simulink model "STM_SIMULINK_BLDC"  (R2022a)
settings: Solver=FixedStepAuto  StartTime=0.0  StopTime=10.0  FixedStep=0.001  RelTol=1e-3  EnableMultiTasking=on
InitFcn:
  | dataType = 'single';
  | 
  | motor.polePairs = 6;
  | motor.base_speed = 4000;
  | motor.base_freq = 266.6667;
  | max_rpm = 1000;
  | Ts = 1e-3;
undefined symbols (not defined in the file or in its folder): DiscIntNeverNeededParam
libraries: mcbcontrolslib x2
settings Model: ExtModeTrigDuration=10  Creator=s269684  LastModifiedBy=s269684
settings OptimizationCC: EnhancedBackFolding=on  PassReuseOutputArgsAs=Individual arguments  ZeroExternalMemoryAtStartup=off  ZeroInternalMemoryAtStartup=off  MaxStackSize=64  OptimizeBlockOrder=speed  DifferentSizesBufferReuse=on  OptimizationCustomize=off  EfficientTunableParamExpr=on
settings DebuggingCC: ParameterTunabilityLossMsg=error
settings HardwareCC: ProdBitPerPointer=32  ProdBitPerSizeT=32  ProdBitPerPtrDiffT=32  ProdLargestAtomicInteger=Long  ProdLargestAtomicFloat=Double  ProdWordSize=32  ProdLongLongMode=on  ProdHWDeviceType=ARM Compatible->ARM Cortex
settings SFSimCC: MATLABDynamicMemAlloc=off
settings RTWCC: SystemTargetFile=ert.tlc  HardwareBoard=STM32 Nucleo F302R8  TemplateMakefile=ert_default_tmf  Toolchain=GNU Tools for ARM Embedded Processors
settings CodeAppCC: ForceParamTrailComments=on  IgnoreCustomStorageClasses=off  OperatorAnnotations=on  SimulinkDataObjDesc=on  SFDataObjDesc=on  InsertBlockDesc=on
settings ERTTargetCC: ExtModeTransport=3  ExtModeStaticAlloc=on  ExtModeStaticAllocSize=1000  ExtModeMexFile=ext_xcp  ExtModeIntrfLevel=Level2 - Open

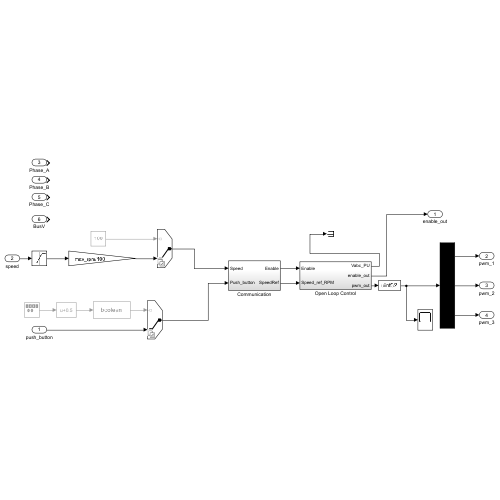
[thumbnail: Simulink's stored preview of the top-level diagram]
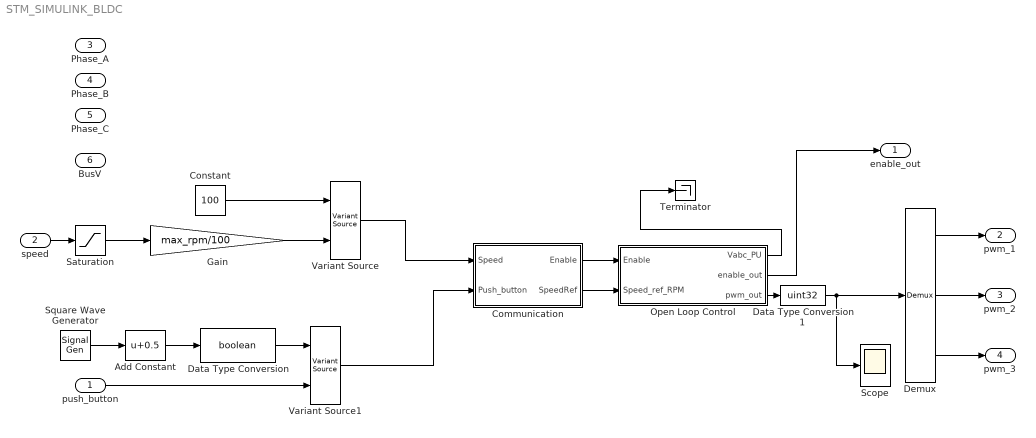
== system STM_SIMULINK_BLDC ==
  push_button : Inport  OutDataTypeStr=boolean
  speed : Inport  Port=2  OutDataTypeStr=uint16
  Phase_A : Inport  Port=3  OutDataTypeStr=uint16
  Phase_B : Inport  Port=4  OutDataTypeStr=uint16
  Phase_C : Inport  Port=5  OutDataTypeStr=uint16
  BusV : Inport  Port=6  OutDataTypeStr=uint16
  Add Constant : Bias  Bias=0.5  SaturateOnIntegerOverflow=off
  Communication : Subsystem
  Constant : Constant  Value=100  OutDataTypeStr=dataType
  Data Type Conversion : DataTypeConversion  OutDataTypeStr=boolean  SaturateOnIntegerOverflow=off  RndMeth=Floor
  Data Type Conversion1 : DataTypeConversion  OutDataTypeStr=uint32  SaturateOnIntegerOverflow=off  RndMeth=Floor
  Demux : Demux  Outputs=3
  Gain : Gain  Gain=max_rpm/100
  Open Loop Control : Subsystem
  Saturation : Saturate  UpperLimit=100  LowerLimit=0
  Scope : Scope
  Square Wave Generator : SignalGenerator  WaveForm=square  Amplitude=0.5  Frequency=0.5
  Terminator : Terminator
  Variant Source : VariantSource  VariantControlMode=sim codegen switching
  Variant Source1 : VariantSource  VariantControlMode=sim codegen switching
  enable_out : Outport
  pwm_1 : Outport  Port=2
  pwm_2 : Outport  Port=3
  pwm_3 : Outport  Port=4
  wires:
  Communication/2(SpeedRef) -> Open Loop Control/2(Speed_ref_RPM)
  Add Constant/1 -> Data Type Conversion/1
  Square Wave Generator/1 -> Add Constant/1
  Variant Source1/1 -> Communication/2(Push_button)
  Data Type Conversion/1 -> Variant Source1/1
  Saturation/1 -> Gain/1
  Open Loop Control/2(enable_out) -> enable_out/1
  speed/1 -> Saturation/1
  Demux/2 -> pwm_2/1
  Demux/1 -> pwm_1/1
  Open Loop Control/1(Vabc_PU) -> Terminator/1
  Communication/1(Enable) -> Open Loop Control/1(Enable)
  push_button/1 -> Variant Source1/2
  Variant Source/1 -> Communication/1(Speed)
  Data Type Conversion1/1 -> Scope/1, Demux/1
  Constant/1 -> Variant Source/1
  Open Loop Control/3(pwm_out) -> Data Type Conversion1/1
  Gain/1 -> Variant Source/2
  Demux/3 -> pwm_3/1

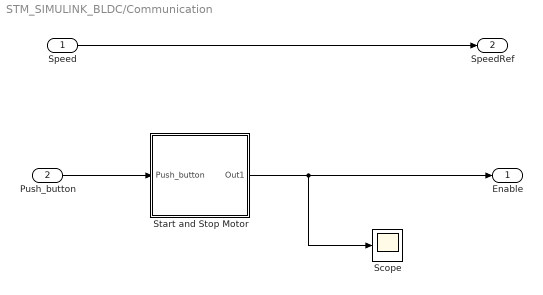
== system STM_SIMULINK_BLDC/Communication ==
  Speed : Inport
  Push_button : Inport  Port=2
  Scope : Scope
  Start and Stop Motor : Subsystem  TreatAsAtomicUnit=on  SystemSampleTime=1e-3
  Enable : Outport
  SpeedRef : Outport  Port=2  VectorParamsAs1DForOutWhenUnconnected=off
  wires:
  Speed/1 -> SpeedRef/1
  Start and Stop Motor/1(Out1) -> Scope/1, Enable/1
  Push_button/1 -> Start and Stop Motor/1(Push_button)

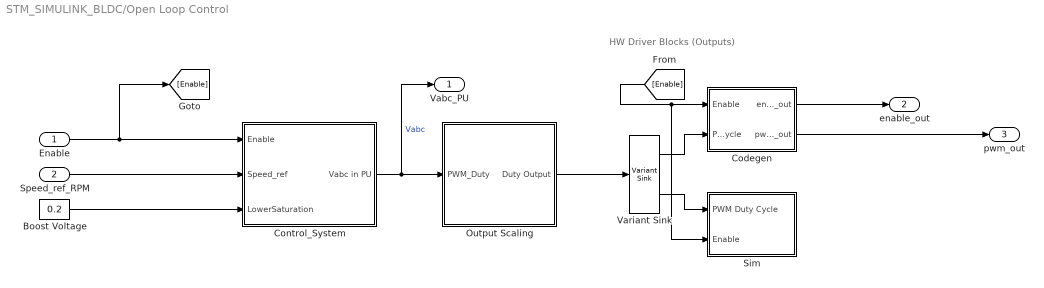
== system STM_SIMULINK_BLDC/Open Loop Control ==
  note: HW Driver Blocks (Outputs)
  Enable : Inport
  Speed_ref_RPM : Inport  Port=2
  Boost Voltage : Constant  Value=0.2  OutDataTypeStr=single
  Codegen : Subsystem
      settings: RTWSystemCode=Nonreusable function
  Control_System : Subsystem
      settings: RTWSystemCode=Nonreusable function
  Output Scaling : Subsystem
      settings: RTWSystemCode=Nonreusable function
  Sim : Subsystem
  Variant Sink : VariantSink  VariantControlMode=sim codegen switching
  Vabc_PU : Outport  VectorParamsAs1DForOutWhenUnconnected=off
  enable_out : Outport  Port=2
  pwm_out : Outport  Port=3
  wires:
  Control_System/1(Vabc in PU) -> Output Scaling/1(PWM_Duty), Vabc_PU/1  "Vabc"
  Boost Voltage/1 -> Control_System/3(LowerSaturation)
  Enable/1 -> [Enable], Control_System/1(Enable)
  Speed_ref_RPM/1 -> Control_System/2(Speed_ref)
  [Enable] -> Sim/2(Enable), Codegen/1(Enable)
  Variant Sink/1 -> Codegen/2(PWM Duty Cycle)
  Variant Sink/2 -> Sim/1(PWM Duty Cycle)
  Output Scaling/1(Duty Output) -> Variant Sink/1
  Codegen/1(enable_out) -> enable_out/1
  Codegen/2(pwm_out) -> pwm_out/1

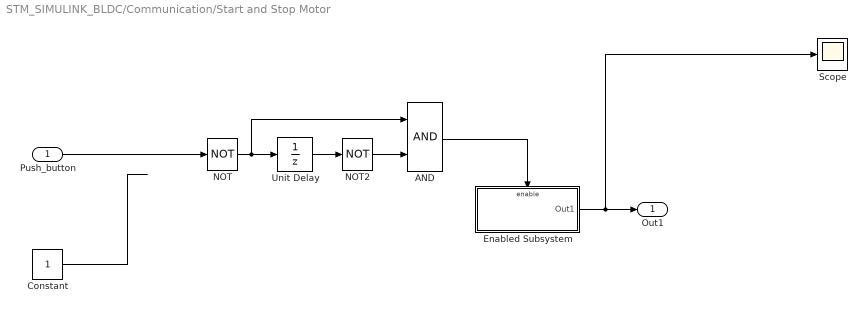
== system STM_SIMULINK_BLDC/Communication/Start and Stop Motor ==
  Push_button : Inport
  AND : Logic  AllPortsSameDT=off  OutDataTypeStr=boolean
  Constant : Constant  SampleTime=-1
  Enabled Subsystem : Subsystem  TreatAsAtomicUnit=on
  NOT : Logic  Operator=NOT  IconShape=distinctive  AllPortsSameDT=off  OutDataTypeStr=boolean
  NOT2 : Logic  Operator=NOT  IconShape=distinctive  AllPortsSameDT=off  OutDataTypeStr=boolean
  Scope : Scope
  Unit Delay : UnitDelay  InitialCondition=false  SampleTime=-1  HasFrameUpgradeWarning=on
  Out1 : Outport
  wires:
  Enabled Subsystem/1(Out1) -> Scope/1, Out1/1
  AND/1 -> Enabled Subsystem/Enable
  Push_button/1 -> NOT/1
  Unit Delay/1 -> NOT2/1
  NOT2/1 -> AND/2
  NOT/1 -> Unit Delay/1, AND/1
  Constant/1 -> ?

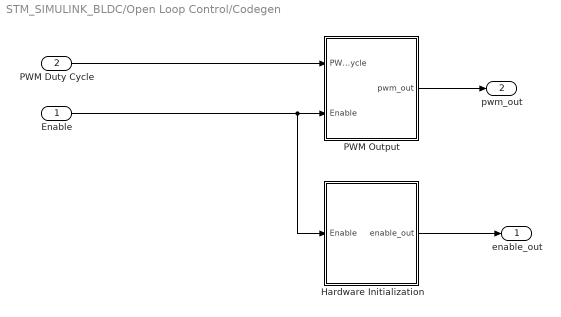
== system STM_SIMULINK_BLDC/Open Loop Control/Codegen ==
  Enable : Inport
  PWM Duty Cycle : Inport  Port=2
  Hardware Initialization : Subsystem
      settings: RTWSystemCode=Nonreusable function
  PWM Output : Subsystem
      settings: RTWSystemCode=Nonreusable function
  enable_out : Outport
  pwm_out : Outport  Port=2
  wires:
  PWM Duty Cycle/1 -> PWM Output/1(PWM Duty Cycle)
  Enable/1 -> Hardware Initialization/1(Enable), PWM Output/2(Enable)
  Hardware Initialization/1(enable_out) -> enable_out/1
  PWM Output/1(pwm_out) -> pwm_out/1

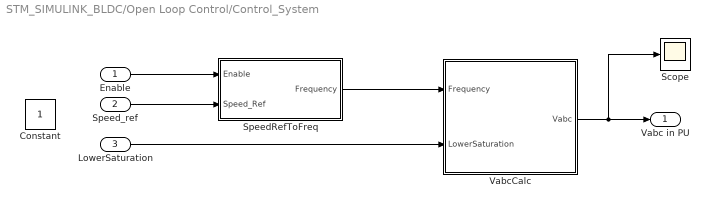
== system STM_SIMULINK_BLDC/Open Loop Control/Control_System ==
  Enable : Inport
  Speed_ref : Inport  Port=2
  LowerSaturation : Inport  Port=3
  Constant : Constant
  Scope : Scope
  SpeedRefToFreq : Subsystem
  VabcCalc : Subsystem
  Vabc in PU : Outport  VectorParamsAs1DForOutWhenUnconnected=off
  wires:
  Speed_ref/1 -> SpeedRefToFreq/2(Speed_Ref)
  SpeedRefToFreq/1(Frequency) -> VabcCalc/1(Frequency)
  LowerSaturation/1 -> VabcCalc/2(LowerSaturation)
  Enable/1 -> SpeedRefToFreq/1(Enable)
  VabcCalc/1(Vabc) -> Scope/1, Vabc in PU/1

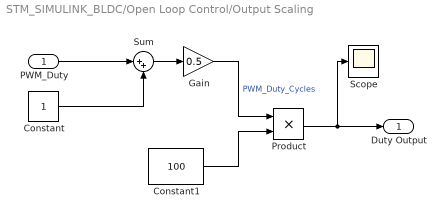
== system STM_SIMULINK_BLDC/Open Loop Control/Output Scaling ==
  PWM_Duty : Inport
  Constant : Constant  OutDataTypeStr=dataType
  Constant1 : Constant  Value=100  OutDataTypeStr=dataType
  Gain : Gain  Gain=0.5  RndMeth=Simplest  OutDataTypeStr=Inherit: Same as input
  Product : Product  RndMeth=Simplest  OutDataTypeStr=Inherit: Same as first input
  Scope : Scope
  Sum : Sum  Inputs=|++
  Duty Output : Outport
  wires:
  Product/1 -> Scope/1, Duty Output/1
  Constant1/1 -> Product/2
  PWM_Duty/1 -> Sum/1
  Constant/1 -> Sum/2
  Sum/1 -> Gain/1
  Gain/1 -> Product/1  "PWM_Duty_Cycles"

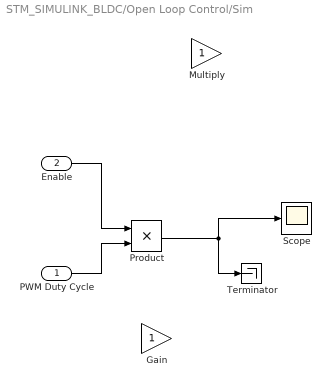
== system STM_SIMULINK_BLDC/Open Loop Control/Sim ==
  PWM Duty Cycle : Inport
  Enable : Inport  Port=2
  Gain : Gain
  Multiply : Gain
  Product : Product
  Scope : Scope
  Terminator : Terminator
  wires:
  Product/1 -> Terminator/1, Scope/1
  Enable/1 -> Product/1
  PWM Duty Cycle/1 -> Product/2

== system STM_SIMULINK_BLDC/Communication/Start and Stop Motor/Enabled Subsystem ==
  Enable : EnablePort
  NOT : Logic  Operator=NOT  IconShape=distinctive  AllPortsSameDT=off  OutDataTypeStr=boolean
  Unit Delay : UnitDelay  InitialCondition=true  SampleTime=-1  HasFrameUpgradeWarning=on
  Out1 : Outport
  wires:
  Unit Delay/1 -> NOT/1, Out1/1
  NOT/1 -> Unit Delay/1

== system STM_SIMULINK_BLDC/Open Loop Control/Codegen/Hardware Initialization ==
  Enable : Inport
  Constant1 : Constant  Value=0.5  OutDataTypeStr=uint16
  NOT : Logic  Operator=NOT  IconShape=distinctive  AllPortsSameDT=off  OutDataTypeStr=boolean
  Switch : Switch  Criteria=u2 > Threshold  OutDataTypeStr=boolean  RndMeth=Simplest  SaturateOnIntegerOverflow=off  InputSameDT=off
  enable_out : Outport
  wires:
  Enable/1 -> NOT/1, Switch/1
  Constant1/1 -> Switch/2
  NOT/1 -> Switch/3
  Switch/1 -> enable_out/1

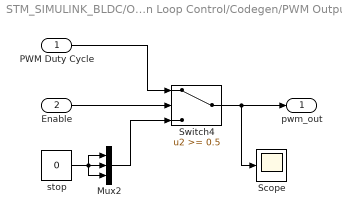
== system STM_SIMULINK_BLDC/Open Loop Control/Codegen/PWM Output ==
  PWM Duty Cycle : Inport
  Enable : Inport  Port=2
  Mux2 : Mux  Inputs=3
  Scope : Scope
  Switch4 : Switch  Threshold=0.5  RndMeth=Simplest  SaturateOnIntegerOverflow=off  InputSameDT=off
  stop : Constant  Value=0  OutDataTypeStr=single
  pwm_out : Outport
  wires:
  stop/1 -> Mux2/3, Mux2/2, Mux2/1
  PWM Duty Cycle/1 -> Switch4/1
  Mux2/1 -> Switch4/3
  Enable/1 -> Switch4/2
  Switch4/1 -> Scope/1, pwm_out/1

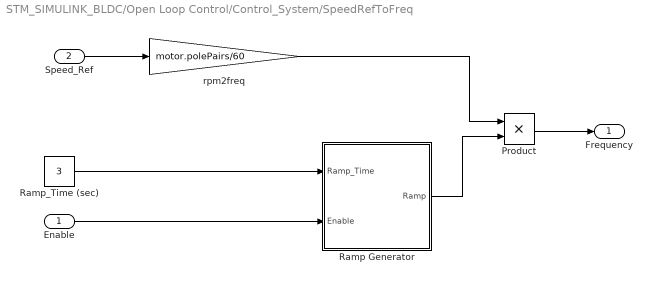
== system STM_SIMULINK_BLDC/Open Loop Control/Control_System/SpeedRefToFreq ==
  Enable : Inport
  Speed_Ref : Inport  Port=2
  Product : Product  RndMeth=Simplest  OutDataTypeStr=Inherit: Same as first input
  Ramp Generator : Subsystem
  Ramp_Time (sec) : Constant  Value=3  OutDataTypeStr=dataType  SampleTime=-1
  rpm2freq : Gain  Gain=motor.polePairs/60  OutDataTypeStr=dataType  RndMeth=Simplest
  Frequency : Outport
  wires:
  Product/1 -> Frequency/1
  Ramp Generator/1(Ramp) -> Product/2
  Ramp_Time (sec)/1 -> Ramp Generator/1(Ramp_Time)
  Enable/1 -> Ramp Generator/2(Enable)
  Speed_Ref/1 -> rpm2freq/1
  rpm2freq/1 -> Product/1

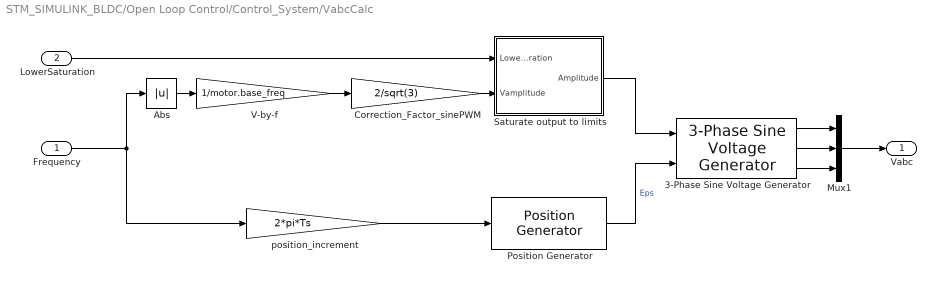
== system STM_SIMULINK_BLDC/Open Loop Control/Control_System/VabcCalc ==
  Frequency : Inport
  LowerSaturation : Inport  Port=2
  3-Phase Sine Voltage Generator : mcbcontrolslib/3-Phase Sine Voltage Generator  AngleInput=Radians  N_points=1024
      settings: SourceProductBaseCode=MT
  Abs : Abs  RndMeth=Simplest  SaturateOnIntegerOverflow=off
  Correction_Factor_sinePWM : Gain  Gain=2/sqrt(3)  RndMeth=Simplest  OutDataTypeStr=Inherit: Same as input
  Mux1 : Mux  Inputs=3
  Position Generator : mcbcontrolslib/Position Generator  AngleOutput=Radians  ThetaSource=External  ThetaInput=5e-4  DataType=double  ExternalReset=none  Offset=0
      settings: SourceProductBaseCode=MT
  Saturate output to limits : Subsystem
  V-by-f : Gain  Gain=1/motor.base_freq  RndMeth=Simplest  OutDataTypeStr=Inherit: Same as input
  position_increment : Gain  Gain=2*pi*Ts  RndMeth=Simplest  OutDataTypeStr=Inherit: Same as input
  Vabc : Outport
  wires:
  position_increment/1 -> Position Generator/1
  3-Phase Sine Voltage Generator/3 -> Mux1/3
  3-Phase Sine Voltage Generator/2 -> Mux1/2
  V-by-f/1 -> Correction_Factor_sinePWM/1
  3-Phase Sine Voltage Generator/1 -> Mux1/1
  Correction_Factor_sinePWM/1 -> Saturate output to limits/2(Vamplitude)
  Mux1/1 -> Vabc/1
  LowerSaturation/1 -> Saturate output to limits/1(Lower Saturation)
  Saturate output to limits/1(Amplitude) -> 3-Phase Sine Voltage Generator/1
  Position Generator/1 -> 3-Phase Sine Voltage Generator/2  "Eps"
  Abs/1 -> V-by-f/1
  Frequency/1 -> Abs/1, position_increment/1

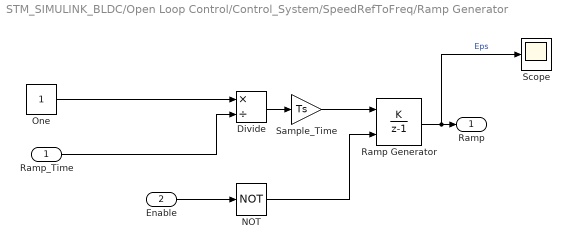
== system STM_SIMULINK_BLDC/Open Loop Control/Control_System/SpeedRefToFreq/Ramp Generator ==
  Ramp_Time : Inport
  Enable : Inport  Port=2
  Divide : Product  Inputs=*/  RndMeth=Simplest  OutDataTypeStr=Inherit: Same as first input
  NOT : Logic  Operator=NOT  IconShape=distinctive  AllPortsSameDT=off  OutDataTypeStr=boolean
  One : Constant  OutDataTypeStr=dataType  SampleTime=-1
  Ramp Generator : DiscreteIntegrator  IntegratorMethod=Accumulation: Forward Euler  gainval=1  ExternalReset=either  SampleTime=-1  OutDataTypeStr=dataType  RndMeth=Simplest  LimitOutput=on  UpperSaturationLimit=1  LowerSaturationLimit=0  ICPrevOutput=DiscIntNeverNeededParam  ICPrevScaledInput=DiscIntNeverNeededParam
  Sample_Time : Gain  Gain=Ts  RndMeth=Simplest  OutDataTypeStr=Inherit: Same as input
  Scope : Scope
  Ramp : Outport
  wires:
  Divide/1 -> Sample_Time/1
  Ramp Generator/1 -> Scope/1, Ramp/1  "Eps"
  Sample_Time/1 -> Ramp Generator/1
  One/1 -> Divide/1
  Ramp_Time/1 -> Divide/2
  Enable/1 -> NOT/1
  NOT/1 -> Ramp Generator/2

== system STM_SIMULINK_BLDC/Open Loop Control/Control_System/VabcCalc/Saturate output to limits ==
  Lower Saturation : Inport
  Vamplitude : Inport  Port=2
  Relational Operator : RelationalOperator  Operator=>  OutDataTypeStr=boolean  RndMeth=Simplest  InputSameDT=off
  Saturation : Saturate  UpperLimit=0.95  LowerLimit=0  RndMeth=Simplest
  Switch : Switch  Criteria=u2 > Threshold  SaturateOnIntegerOverflow=off  InputSameDT=off
  Amplitude : Outport
  wires:
  Saturation/1 -> Amplitude/1
  Switch/1 -> Saturation/1
  Relational Operator/1 -> Switch/2
  Lower Saturation/1 -> Switch/3, Relational Operator/2
  Vamplitude/1 -> Switch/1, Relational Operator/1
